simulink model "MyPowerTrain_RTW"  (R2022b)
settings: Solver=ode1  StartTime=0.0  StopTime=inf  FixedStep=0.0002  RelTol=1e-3
PreLoadFcn:
  | vehicle = 'Car'; if ~length(which('cmself')), cmenv; end
  | MyPowerTrain_RTW_bus
InitFcn:
  | vehicle = 'Car'; if ~length(which('cmself')), cmenv; end
  | MyPowerTrain_RTW_bus
libraries: simulink x4, CarMaker4SL x3
Description:
  | CarMaker Plug-in Model Target
settings Model: Creator=developer  LastModifiedBy=developer
settings RTWCC: Description=CarMaker Plug-in Model Target  SystemTargetFile=CarMaker.tlc  TemplateMakefile=CarMaker_unix-win64.tmf  CustomSourceCode="#include \"SimCore.h\""
settings CodeAppCC: MaxIdLength=127
settings STFCustomTargetCC: TargetLangStandard=C99 (ISO)  CombineOutputUpdateFcns=on  CodeInterfacePackaging=Reusable function  GenerateAllocFcn=on  SystemTargetFile=CarMaker.tlc
settings GRTTargetCC: ParMdlRefBuildCompliant=off  CompOptLevelCompliant=off  ConcurrentExecutionCompliant=off  MatFileLogging=off  CodeInterfacePackaging=Reusable function  CPPClassGenCompliant=off  GenerateAllocFcn=on  UseToolchainInfoCompliant=off

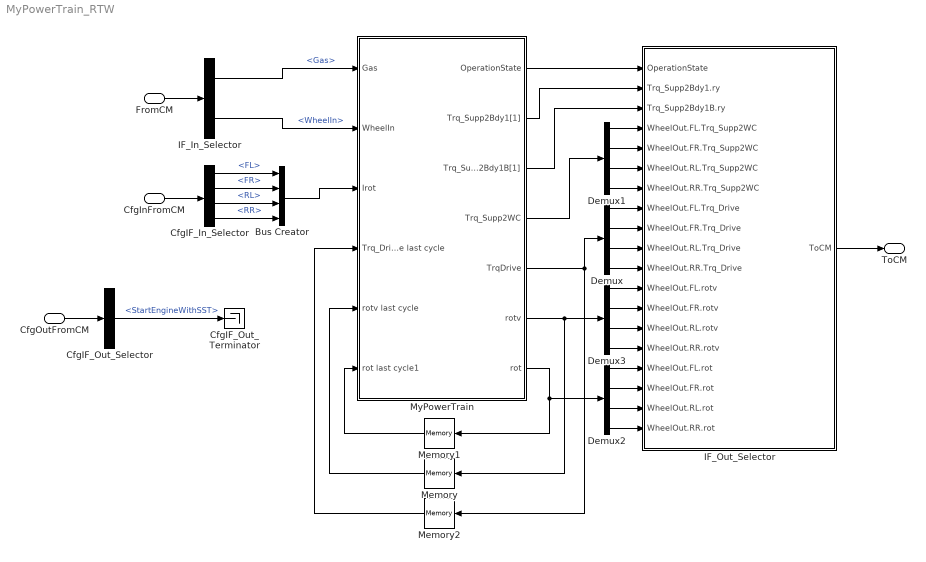
== system MyPowerTrain_RTW ==
  FromCM : Inport  OutDataTypeStr=Bus: cmPowerTrainIn
  CfgInFromCM : Inport  Port=2  OutDataTypeStr=Bus: cmPowerTrainCfgIn
  CfgOutFromCM : Inport  Port=3  OutDataTypeStr=Bus: cmPowerTrainCfgOut
  Bus Creator : BusCreator  Inputs=4
  CfgIF_In_Selector : BusSelector  OutputSignals=Wheel_Iyy.FL,Wheel_Iyy.FR,Wheel_Iyy.RL,Wheel_Iyy.RR
  CfgIF_Out_Selector : BusSelector  OutputSignals=StartEngineWithSST
  CfgIF_Out_Terminator : Terminator
  Demux{,1..3} (4 alike) : Demux
  IF_In_Selector : BusSelector  OutputSignals=Gas,WheelIn
  IF_Out_Selector : Subsystem  mask(Signal Selection){}
      mask help: Signal Selection Block
      settings: OpenFcn=cmSignalSelect('SignalSelection_CB',gcb)
  Memory : Memory
  Memory1 : Memory
  Memory2 : Memory
  MyPowerTrain : Subsystem
  ToCM : Outport  OutDataTypeStr=Bus: cmPowerTrainOut
  wires:
  FromCM/1 -> IF_In_Selector/1
  IF_Out_Selector/1(ToCM) -> ToCM/1
  CfgInFromCM/1 -> CfgIF_In_Selector/1
  CfgOutFromCM/1 -> CfgIF_Out_Selector/1
  CfgIF_Out_Selector/1 -> CfgIF_Out_Terminator/1  "<StartEngineWithSST>"
  Demux2/1 -> IF_Out_Selector/16(WheelOut.FL.rot)
  CfgIF_In_Selector/4 -> Bus Creator/4  "<RR>"
  Memory/1 -> MyPowerTrain/5(rotv last cycle)
  Demux3/4 -> IF_Out_Selector/15(WheelOut.RR.rotv)
  MyPowerTrain/2(Trq_Supp2Bdy1[1]) -> IF_Out_Selector/2(Trq_Supp2Bdy1.ry)
  Demux2/4 -> IF_Out_Selector/19(WheelOut.RR.rot)
  Demux1/1 -> IF_Out_Selector/4(WheelOut.FL.Trq_Supp2WC)
  Memory1/1 -> MyPowerTrain/6(rot last cycle1)
  CfgIF_In_Selector/1 -> Bus Creator/1  "<FL>"
  Demux1/3 -> IF_Out_Selector/6(WheelOut.RL.Trq_Supp2WC)
  MyPowerTrain/6(rotv) -> Demux3/1, Memory/1
  Demux/4 -> IF_Out_Selector/11(WheelOut.RR.Trq_Drive)
  Demux/2 -> IF_Out_Selector/9(WheelOut.FR.Trq_Drive)
  MyPowerTrain/7(rot) -> Demux2/1, Memory1/1
  IF_In_Selector/1 -> MyPowerTrain/1(Gas)  "<Gas>"
  Demux/3 -> IF_Out_Selector/10(WheelOut.RL.Trq_Drive)
  CfgIF_In_Selector/3 -> Bus Creator/3  "<RL>"
  Demux3/2 -> IF_Out_Selector/13(WheelOut.FR.rotv)
  Memory2/1 -> MyPowerTrain/4(Trq_Drive last cycle)
  Demux3/3 -> IF_Out_Selector/14(WheelOut.RL.rotv)
  MyPowerTrain/5(TrqDrive) -> Demux/1, Memory2/1
  MyPowerTrain/3(Trq_Supp2Bdy1B[1]) -> IF_Out_Selector/3(Trq_Supp2Bdy1B.ry)
  Demux2/3 -> IF_Out_Selector/18(WheelOut.RL.rot)
  Demux1/2 -> IF_Out_Selector/5(WheelOut.FR.Trq_Supp2WC)
  CfgIF_In_Selector/2 -> Bus Creator/2  "<FR>"
  Demux2/2 -> IF_Out_Selector/17(WheelOut.FR.rot)
  Bus Creator/1 -> MyPowerTrain/3(Irot)
  Demux/1 -> IF_Out_Selector/8(WheelOut.FL.Trq_Drive)
  Demux1/4 -> IF_Out_Selector/7(WheelOut.RR.Trq_Supp2WC)
  MyPowerTrain/4(Trq_Supp2WC) -> Demux1/1
  Demux3/1 -> IF_Out_Selector/12(WheelOut.FL.rotv)
  IF_In_Selector/2 -> MyPowerTrain/2(WheelIn)  "<WheelIn>"
  MyPowerTrain/1(OperationState) -> IF_Out_Selector/1(OperationState)

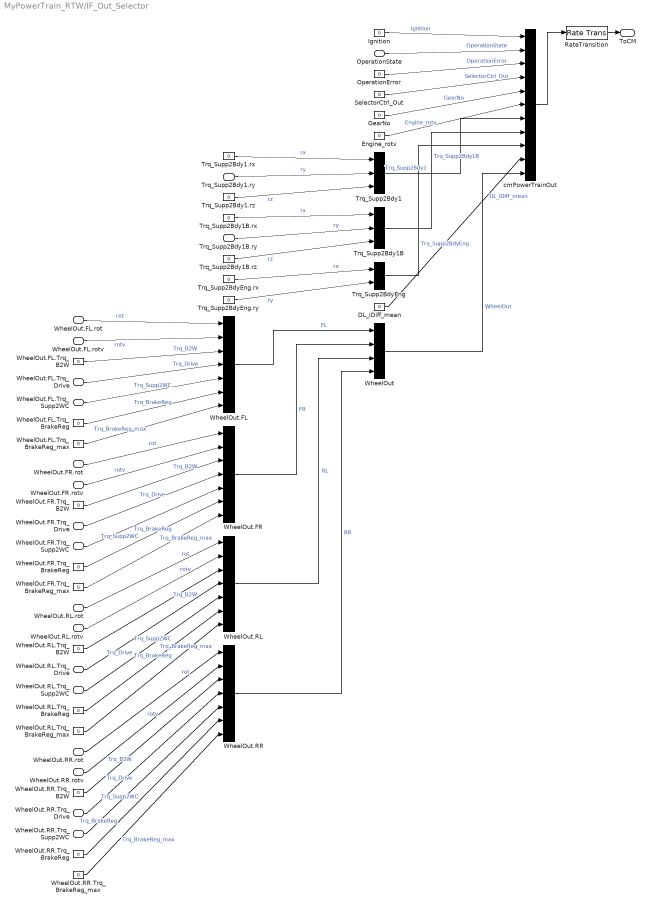
== system MyPowerTrain_RTW/IF_Out_Selector ==
  OperationState : Inport
  Trq_Supp2Bdy1.ry : Inport  Port=2
  Trq_Supp2Bdy1B.ry : Inport  Port=3
  WheelOut.FL.Trq_Supp2WC : Inport  Port=4
  WheelOut.FR.Trq_Supp2WC : Inport  Port=5
  WheelOut.RL.Trq_Supp2WC : Inport  Port=6
  WheelOut.RR.Trq_Supp2WC : Inport  Port=7
  WheelOut.FL.Trq_Drive : Inport  Port=8
  WheelOut.FR.Trq_Drive : Inport  Port=9
  WheelOut.RL.Trq_Drive : Inport  Port=10
  WheelOut.RR.Trq_Drive : Inport  Port=11
  WheelOut.FL.rotv : Inport  Port=12
  WheelOut.FR.rotv : Inport  Port=13
  WheelOut.RL.rotv : Inport  Port=14
  WheelOut.RR.rotv : Inport  Port=15
  WheelOut.FL.rot : Inport  Port=16
  WheelOut.FR.rot : Inport  Port=17
  WheelOut.RL.rot : Inport  Port=18
  WheelOut.RR.rot : Inport  Port=19
  DL_iDiff_mean : Constant  Value=0
  Engine_rotv : Constant  Value=0
  GearNo : Constant  Value=0
  Ignition : Constant  Value=0
  OperationError : Constant  Value=0
  RateTransition : RateTransition  OutPortSampleTime=str2num(get_param(bdroot,'FixedStep'))
  SelectorCtrl_Out : Constant  Value=0
  Trq_Supp2Bdy1 : BusCreator  Inputs=3
  Trq_Supp2Bdy1.rx : Constant  Value=0
  Trq_Supp2Bdy1.rz : Constant  Value=0
  Trq_Supp2Bdy1B : BusCreator  Inputs=3
  Trq_Supp2Bdy1B.rx : Constant  Value=0
  Trq_Supp2Bdy1B.rz : Constant  Value=0
  Trq_Supp2BdyEng : BusCreator  Inputs=2
  Trq_Supp2BdyEng.rx : Constant  Value=0
  Trq_Supp2BdyEng.ry : Constant  Value=0
  WheelOut : BusCreator  Inputs=4
  WheelOut.FL : BusCreator  Inputs=7
  WheelOut.FL.Trq_B2W : Constant  Value=0
  WheelOut.FL.Trq_BrakeReg : Constant  Value=0
  WheelOut.FL.Trq_BrakeReg_max : Constant  Value=0
  WheelOut.FR : BusCreator  Inputs=7
  WheelOut.FR.Trq_B2W : Constant  Value=0
  WheelOut.FR.Trq_BrakeReg : Constant  Value=0
  WheelOut.FR.Trq_BrakeReg_max : Constant  Value=0
  WheelOut.RL : BusCreator  Inputs=7
  WheelOut.RL.Trq_B2W : Constant  Value=0
  WheelOut.RL.Trq_BrakeReg : Constant  Value=0
  WheelOut.RL.Trq_BrakeReg_max : Constant  Value=0
  WheelOut.RR : BusCreator  Inputs=7
  WheelOut.RR.Trq_B2W : Constant  Value=0
  WheelOut.RR.Trq_BrakeReg : Constant  Value=0
  WheelOut.RR.Trq_BrakeReg_max : Constant  Value=0
  cmPowerTrainOut : BusCreator  Inputs=11
  ToCM : Outport
  wires:
  RateTransition/1 -> ToCM/1
  cmPowerTrainOut/1 -> RateTransition/1
  Ignition/1 -> cmPowerTrainOut/1  "Ignition"
  OperationError/1 -> cmPowerTrainOut/3  "OperationError"
  SelectorCtrl_Out/1 -> cmPowerTrainOut/4  "SelectorCtrl_Out"
  GearNo/1 -> cmPowerTrainOut/5  "GearNo"
  Engine_rotv/1 -> cmPowerTrainOut/6  "Engine_rotv"
  Trq_Supp2Bdy1/1 -> cmPowerTrainOut/7  "Trq_Supp2Bdy1"
  Trq_Supp2Bdy1.rx/1 -> Trq_Supp2Bdy1/1  "rx"
  Trq_Supp2Bdy1.rz/1 -> Trq_Supp2Bdy1/3  "rz"
  Trq_Supp2Bdy1B/1 -> cmPowerTrainOut/8  "Trq_Supp2Bdy1B"
  Trq_Supp2Bdy1B.rx/1 -> Trq_Supp2Bdy1B/1  "rx"
  Trq_Supp2Bdy1B.rz/1 -> Trq_Supp2Bdy1B/3  "rz"
  Trq_Supp2BdyEng/1 -> cmPowerTrainOut/9  "Trq_Supp2BdyEng"
  Trq_Supp2BdyEng.rx/1 -> Trq_Supp2BdyEng/1  "rx"
  Trq_Supp2BdyEng.ry/1 -> Trq_Supp2BdyEng/2  "ry"
  DL_iDiff_mean/1 -> cmPowerTrainOut/10  "DL_iDiff_mean"
  WheelOut/1 -> cmPowerTrainOut/11  "WheelOut"
  WheelOut.FL/1 -> WheelOut/1  "FL"
  WheelOut.FL.Trq_B2W/1 -> WheelOut.FL/3  "Trq_B2W"
  WheelOut.FL.Trq_BrakeReg/1 -> WheelOut.FL/6  "Trq_BrakeReg"
  WheelOut.FL.Trq_BrakeReg_max/1 -> WheelOut.FL/7  "Trq_BrakeReg_max"
  WheelOut.FR/1 -> WheelOut/2  "FR"
  WheelOut.FR.Trq_B2W/1 -> WheelOut.FR/3  "Trq_B2W"
  WheelOut.FR.Trq_BrakeReg/1 -> WheelOut.FR/6  "Trq_BrakeReg"
  WheelOut.FR.Trq_BrakeReg_max/1 -> WheelOut.FR/7  "Trq_BrakeReg_max"
  WheelOut.RL/1 -> WheelOut/3  "RL"
  WheelOut.RL.Trq_B2W/1 -> WheelOut.RL/3  "Trq_B2W"
  WheelOut.RL.Trq_BrakeReg/1 -> WheelOut.RL/6  "Trq_BrakeReg"
  WheelOut.RL.Trq_BrakeReg_max/1 -> WheelOut.RL/7  "Trq_BrakeReg_max"
  WheelOut.RR/1 -> WheelOut/4  "RR"
  WheelOut.RR.Trq_B2W/1 -> WheelOut.RR/3  "Trq_B2W"
  WheelOut.RR.Trq_BrakeReg/1 -> WheelOut.RR/6  "Trq_BrakeReg"
  WheelOut.RR.Trq_BrakeReg_max/1 -> WheelOut.RR/7  "Trq_BrakeReg_max"
  OperationState/1 -> cmPowerTrainOut/2  "OperationState"
  Trq_Supp2Bdy1.ry/1 -> Trq_Supp2Bdy1/2  "ry"
  Trq_Supp2Bdy1B.ry/1 -> Trq_Supp2Bdy1B/2  "ry"
  WheelOut.FL.Trq_Supp2WC/1 -> WheelOut.FL/5  "Trq_Supp2WC"
  WheelOut.FR.Trq_Supp2WC/1 -> WheelOut.FR/5  "Trq_Supp2WC"
  WheelOut.RL.Trq_Supp2WC/1 -> WheelOut.RL/5  "Trq_Supp2WC"
  WheelOut.RR.Trq_Supp2WC/1 -> WheelOut.RR/5  "Trq_Supp2WC"
  WheelOut.FL.Trq_Drive/1 -> WheelOut.FL/4  "Trq_Drive"
  WheelOut.FR.Trq_Drive/1 -> WheelOut.FR/4  "Trq_Drive"
  WheelOut.RL.Trq_Drive/1 -> WheelOut.RL/4  "Trq_Drive"
  WheelOut.RR.Trq_Drive/1 -> WheelOut.RR/4  "Trq_Drive"
  WheelOut.FL.rotv/1 -> WheelOut.FL/2  "rotv"
  WheelOut.FR.rotv/1 -> WheelOut.FR/2  "rotv"
  WheelOut.RL.rotv/1 -> WheelOut.RL/2  "rotv"
  WheelOut.RR.rotv/1 -> WheelOut.RR/2  "rotv"
  WheelOut.FL.rot/1 -> WheelOut.FL/1  "rot"
  WheelOut.FR.rot/1 -> WheelOut.FR/1  "rot"
  WheelOut.RL.rot/1 -> WheelOut.RL/1  "rot"
  WheelOut.RR.rot/1 -> WheelOut.RR/1  "rot"

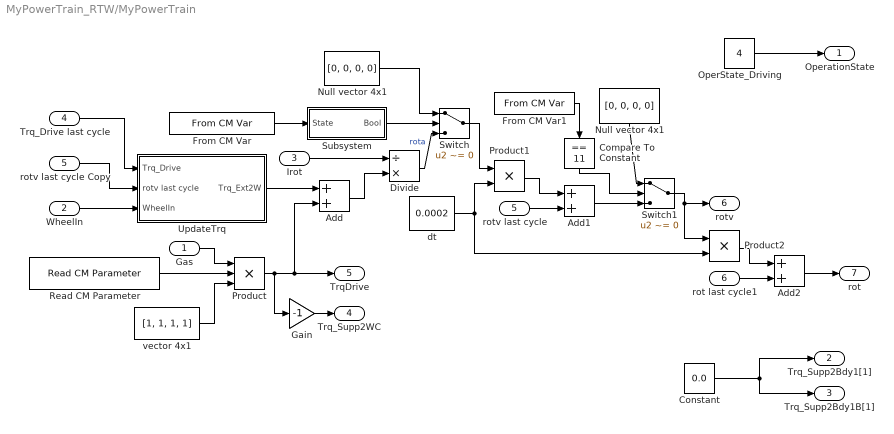
== system MyPowerTrain_RTW/MyPowerTrain ==
  Gas : Inport
  WheelIn : Inport  Port=2
  Irot : Inport  Port=3
  Trq_Drive last cycle : Inport  Port=4
  rotv last cycle : Inport  Port=5
  rot last cycle1 : Inport  Port=6
  Add : Sum
  Add1 : Sum
  Add2 : Sum
  Compare To Constant : simulink/Logic and Bit Operations/Compare To Constant  relop===  const=11  OutDataTypeStr=uint8  ZeroCross=off
  Constant : Constant  Value=0.0
  Divide : Product  Inputs=/*
  From CM Var : CarMaker4SL/From CM Var  xname=SimCore.State
      settings: SourceProductName=CarMaker4SL
  From CM Var1 : CarMaker4SL/From CM Var  xname=SimCore.State
      settings: SourceProductName=CarMaker4SL
  Gain : Gain  Gain=-1
  Null vector 4x1 : Constant  Value=[0, 0, 0, 0]
  "Null vector 4x1 " : Constant  Value=[0, 0, 0, 0]
  OperState_Driving : Constant  Value=4
  Product : Product  Inputs=3  RndMeth=Zero
  Product1 : Product  RndMeth=Zero
  Product2 : Product  RndMeth=Zero
  Read CM Parameter : CarMaker4SL/Read CM Parameter  xfile_type=Vehicle  xfile_instance_vehicle=-  xfile_instance_trailer=1  xfile_instance_general=-  xfile_kind_vehicle=Vehicle  xfile_kind_trailer=Trailer  xfile_kind_general=SimParameters  xfile=Vehicle  xkey=MyPowerTrain.Gas2Trq  xnout=1  xdefaults=[]  xmuxed=on  xstime=Continuous
      settings: SourceProductName=CarMaker4SL
  Subsystem : Subsystem
  Switch : Switch  Criteria=u2 ~= 0  SaturateOnIntegerOverflow=off  InputSameDT=off
  Switch1 : Switch  Criteria=u2 ~= 0  SaturateOnIntegerOverflow=off  InputSameDT=off
  UpdateTrq : Subsystem
  dt : Constant  Value=0.0002
  rotv last cycle Copy : InportShadow  Port=5
  vector 4x1 : Constant  Value=[1, 1, 1, 1]
  OperationState : Outport  VectorParamsAs1DForOutWhenUnconnected=off
  Trq_Supp2Bdy1[1] : Outport  Port=2  VectorParamsAs1DForOutWhenUnconnected=off
  Trq_Supp2Bdy1B[1] : Outport  Port=3  VectorParamsAs1DForOutWhenUnconnected=off
  Trq_Supp2WC : Outport  Port=4  VectorParamsAs1DForOutWhenUnconnected=off
  TrqDrive : Outport  Port=5  VectorParamsAs1DForOutWhenUnconnected=off
  rotv : Outport  Port=6  VectorParamsAs1DForOutWhenUnconnected=off
  rot : Outport  Port=7  VectorParamsAs1DForOutWhenUnconnected=off
  wires:
  OperState_Driving/1 -> OperationState/1
  Product/1 -> Gain/1, TrqDrive/1, Add/2
  Read CM Parameter/1 -> Product/2
  Gas/1 -> Product/1
  vector 4x1/1 -> Product/3
  Gain/1 -> Trq_Supp2WC/1
  Add/1 -> Divide/2
  Add2/1 -> rot/1
  rotv last cycle/1 -> Add1/2
  dt/1 -> Product1/2, Product2/2
  Product1/1 -> Add1/1
  Product2/1 -> Add2/1
  Switch/1 -> Product1/1
  Divide/1 -> Switch/3  "rota"
  Null vector 4x1/1 -> Switch/1
  Subsystem/1(Bool) -> Switch/2
  From CM Var/1 -> Subsystem/1(State)
  Add1/1 -> Switch1/3
  Switch1/1 -> rotv/1, Product2/1
  "Null vector 4x1 "/1 -> Switch1/1
  From CM Var1/1 -> Compare To Constant/1
  Compare To Constant/1 -> Switch1/2
  Constant/1 -> Trq_Supp2Bdy1[1]/1, Trq_Supp2Bdy1B[1]/1
  rot last cycle1/1 -> Add2/2
  Irot/1 -> Divide/1
  UpdateTrq/1(Trq_Ext2W) -> Add/1
  Trq_Drive last cycle/1 -> UpdateTrq/1(Trq_Drive)
  rotv last cycle Copy/1 -> UpdateTrq/2(rotv last cycle)
  WheelIn/1 -> UpdateTrq/3(WheelIn)

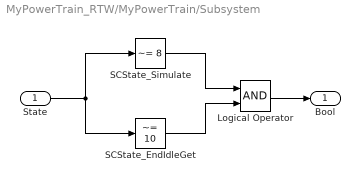
== system MyPowerTrain_RTW/MyPowerTrain/Subsystem ==
  State : Inport
  Logical Operator : Logic  AllPortsSameDT=off  OutDataTypeStr=boolean
  SCState_EndIdleGet : simulink/Logic and Bit Operations/Compare To Constant  relop=~=  const=10  OutDataTypeStr=uint8  ZeroCross=off
  SCState_Simulate : simulink/Logic and Bit Operations/Compare To Constant  relop=~=  const=8  OutDataTypeStr=uint8  ZeroCross=off
  Bool : Outport  VectorParamsAs1DForOutWhenUnconnected=off
  wires:
  Logical Operator/1 -> Bool/1
  SCState_Simulate/1 -> Logical Operator/1
  SCState_EndIdleGet/1 -> Logical Operator/2
  State/1 -> SCState_Simulate/1, SCState_EndIdleGet/1

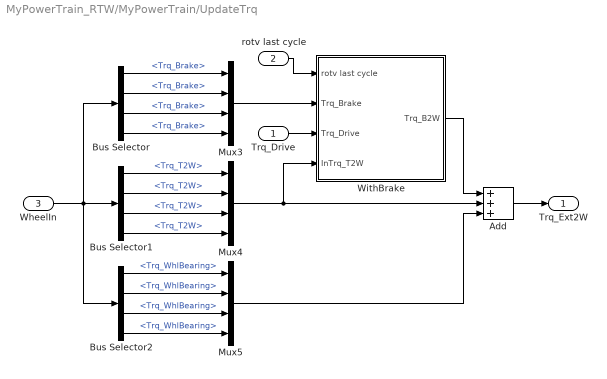
== system MyPowerTrain_RTW/MyPowerTrain/UpdateTrq ==
  Trq_Drive : Inport
  rotv last cycle : Inport  Port=2
  WheelIn : Inport  Port=3
  Add : Sum  Inputs=+++
  Bus Selector : BusSelector  OutputSignals=FL.Trq_Brake,FR.Trq_Brake,RL.Trq_Brake,RR.Trq_Brake
  Bus Selector1 : BusSelector  OutputSignals=FL.Trq_T2W,FR.Trq_T2W,RL.Trq_T2W,RR.Trq_T2W
  Bus Selector2 : BusSelector  OutputSignals=FL.Trq_WhlBearing,FR.Trq_WhlBearing,RL.Trq_WhlBearing,RR.Trq_WhlBearing
  Mux3 : Mux
  Mux4 : Mux
  Mux5 : Mux
  WithBrake : Subsystem
  Trq_Ext2W : Outport  VectorParamsAs1DForOutWhenUnconnected=off
  wires:
  Mux4/1 -> Add/2, WithBrake/4(InTrq_T2W)
  Mux5/1 -> Add/3
  Trq_Drive/1 -> WithBrake/3(Trq_Drive)
  WithBrake/1(Trq_B2W) -> Add/1
  WheelIn/1 -> Bus Selector/1, Bus Selector1/1, Bus Selector2/1
  Bus Selector/1 -> Mux3/1  "<Trq_Brake>"
  Bus Selector/2 -> Mux3/2  "<Trq_Brake>"
  Bus Selector/3 -> Mux3/3  "<Trq_Brake>"
  Bus Selector/4 -> Mux3/4  "<Trq_Brake>"
  Bus Selector1/1 -> Mux4/1  "<Trq_T2W>"
  Bus Selector1/2 -> Mux4/2  "<Trq_T2W>"
  Bus Selector1/3 -> Mux4/3  "<Trq_T2W>"
  Bus Selector1/4 -> Mux4/4  "<Trq_T2W>"
  Bus Selector2/1 -> Mux5/1  "<Trq_WhlBearing>"
  Bus Selector2/2 -> Mux5/2  "<Trq_WhlBearing>"
  Bus Selector2/3 -> Mux5/3  "<Trq_WhlBearing>"
  Bus Selector2/4 -> Mux5/4  "<Trq_WhlBearing>"
  Add/1 -> Trq_Ext2W/1
  Mux3/1 -> WithBrake/2(Trq_Brake)
  rotv last cycle/1 -> WithBrake/1(rotv last cycle)

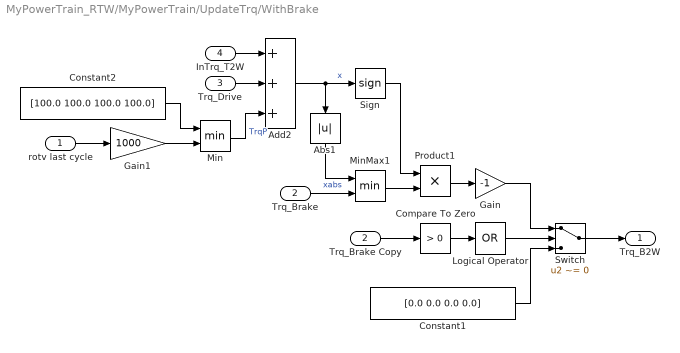
== system MyPowerTrain_RTW/MyPowerTrain/UpdateTrq/WithBrake ==
  rotv last cycle : Inport
  Trq_Brake : Inport  Port=2
  Trq_Drive : Inport  Port=3
  InTrq_T2W : Inport  Port=4
  Abs1 : Abs  SaturateOnIntegerOverflow=off
  Add2 : Sum  Inputs=+++
  Compare To Zero : simulink/Logic and Bit Operations/Compare To Zero  relop=>  OutDataTypeStr=uint8  ZeroCross=off
  Constant1 : Constant  Value=[0.0 0.0 0.0 0.0]
  Constant2 : Constant  Value=[100.0 100.0 100.0 100.0]
  Gain : Gain  Gain=-1
  Gain1 : Gain  Gain=1000
  Logical Operator : Logic  Operator=OR  Inputs=1  AllPortsSameDT=off  OutDataTypeStr=boolean
  Min : MinMax  Inputs=2
  MinMax1 : MinMax  Inputs=2
  Product1 : Product  RndMeth=Zero
  Sign : Signum
  Switch : Switch  Criteria=u2 ~= 0  SaturateOnIntegerOverflow=off  InputSameDT=off
  Trq_Brake Copy : InportShadow  Port=2
  Trq_B2W : Outport  VectorParamsAs1DForOutWhenUnconnected=off
  wires:
  Add2/1 -> Abs1/1, Sign/1  "x"
  Trq_Brake/1 -> MinMax1/2
  Switch/1 -> Trq_B2W/1
  Product1/1 -> Gain/1
  Compare To Zero/1 -> Logical Operator/1
  Abs1/1 -> MinMax1/1  "xabs"
  Constant1/1 -> Switch/3
  Logical Operator/1 -> Switch/2
  MinMax1/1 -> Product1/2
  Sign/1 -> Product1/1
  Trq_Brake Copy/1 -> Compare To Zero/1
  Constant2/1 -> Min/1
  rotv last cycle/1 -> Gain1/1
  Gain1/1 -> Min/2
  Min/1 -> Add2/3  "TrqP"
  InTrq_T2W/1 -> Add2/1
  Trq_Drive/1 -> Add2/2
  Gain/1 -> Switch/1
